simulink model "MIMOWoodBerry"  (R2020b)
settings: Solver=VariableStepAuto  StartTime=0.0  StopTime=400  RelTol=1e-3
values from neighbouring files (symbols this model uses):
  A = sys.A    [MIMOWoodBerry_Continuo.m]    (also in MIMOWoodBerry_Sistema.m)
  B = sys.B    [MIMOWoodBerry_Continuo.m]    (also in MIMOWoodBerry_Sistema.m)
  C = sys.C    [MIMOWoodBerry_Continuo.m]    (also in MIMOWoodBerry_Sistema.m)
  D = sys.D    [MIMOWoodBerry_Continuo.m]    (also in MIMOWoodBerry_Sistema.m)
libraries: cstblocks x1
settings Model: Creator=Sergio  LastModifiedBy=cesar
settings DataIOCC: ReturnWorkspaceOutputs=off
settings DebuggingCC: ArithmeticOperatorsInVariantConditions=warning
settings SFSimCC: SimUseLocalCustomCode=off  CustomCodeUndefinedFunction=UseInterfaceOnly
settings RTWCC: RTWUseLocalCustomCode=off

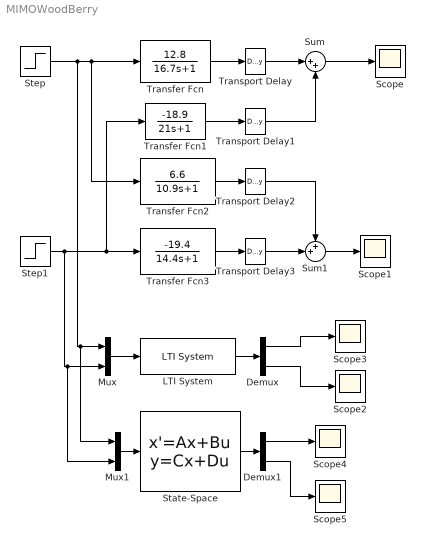
== system MIMOWoodBerry ==
  Demux : Demux  Outputs=2
  Demux1 : Demux  Outputs=2
  LTI System : cstblocks/LTI System  sys=sys  IC=[]
  Mux : Mux  Inputs=2
  Mux1 : Mux  Inputs=2
  Scope{,1..5} (6 alike) : Scope
  State-Space : StateSpace  A=A  B=B  C=C  D=D  InitialCondition=0
  Step : Step  Time=50  SampleTime=0
  Step1 : Step  Time=150  SampleTime=0
  Sum : Sum  Inputs=|++
  Sum1 : Sum  Inputs=++|
  Transfer Fcn : TransferFcn  Numerator=[12.8]  Denominator=[16.7 1]
  Transfer Fcn1 : TransferFcn  Numerator=[-18.9]  Denominator=[21 1]
  Transfer Fcn2 : TransferFcn  Numerator=[6.6]  Denominator=[10.9 1]
  Transfer Fcn3 : TransferFcn  Numerator=[-19.4]  Denominator=[14.4 1]
  Transport Delay : TransportDelay
  Transport Delay1 : TransportDelay  DelayTime=3
  Transport Delay2 : TransportDelay  DelayTime=7
  Transport Delay3 : TransportDelay  DelayTime=3
  wires:
  Step/1 -> Mux1/1, Mux/1, Transfer Fcn2/1, Transfer Fcn/1
  Transfer Fcn/1 -> Transport Delay/1
  Sum/1 -> Scope/1
  Transfer Fcn1/1 -> Transport Delay1/1
  Step1/1 -> Mux1/2, Mux/2, Transfer Fcn1/1, Transfer Fcn3/1
  Transfer Fcn3/1 -> Transport Delay3/1
  Sum1/1 -> Scope1/1
  Transfer Fcn2/1 -> Transport Delay2/1
  Transport Delay/1 -> Sum/1
  Transport Delay1/1 -> Sum/2
  Transport Delay2/1 -> Sum1/1
  Transport Delay3/1 -> Sum1/2
  Mux/1 -> LTI System/1
  LTI System/1 -> Demux/1
  Demux/1 -> Scope3/1
  Demux/2 -> Scope2/1
  State-Space/1 -> Demux1/1
  Mux1/1 -> State-Space/1
  Demux1/1 -> Scope4/1
  Demux1/2 -> Scope5/1
